simulink model "AMCLStateMachine"  (R2016b)
settings: Solver=FixedStepDiscrete  StartTime=0.0  StopTime=inf  FixedStep=0.01  RelTol=1e-3  EnableMultiTasking=on
settings Model: Creator=CHENJH43  LastModifiedBy=CHENJH43
settings SolverCC: AutoInsertRateTranBlk=on
settings DataIOCC: LimitDataPoints=on
settings OptimizationCC: LifeSpan=inf
settings DebuggingCC: AllowSymbolicDim=off  SFUnexpectedBacktrackingDiag=warning  SFNoUnconditionalDefaultTransitionDiag=warning  SFExecutionAtInitializationDiag=none
settings GRTTargetCC: TargetLangStandard=C89/C90 (ANSI)  GeneratePreprocessorConditionals=Disable all
settings ConfigComp: CovMetricSettings=dw  CovHtmlReporting=on  CovSaveCumulativeToWorkspaceVar=on  CovSaveSingleToWorkspaceVar=on  CovExternalEMLEnable=off  CovSFcnEnable=off

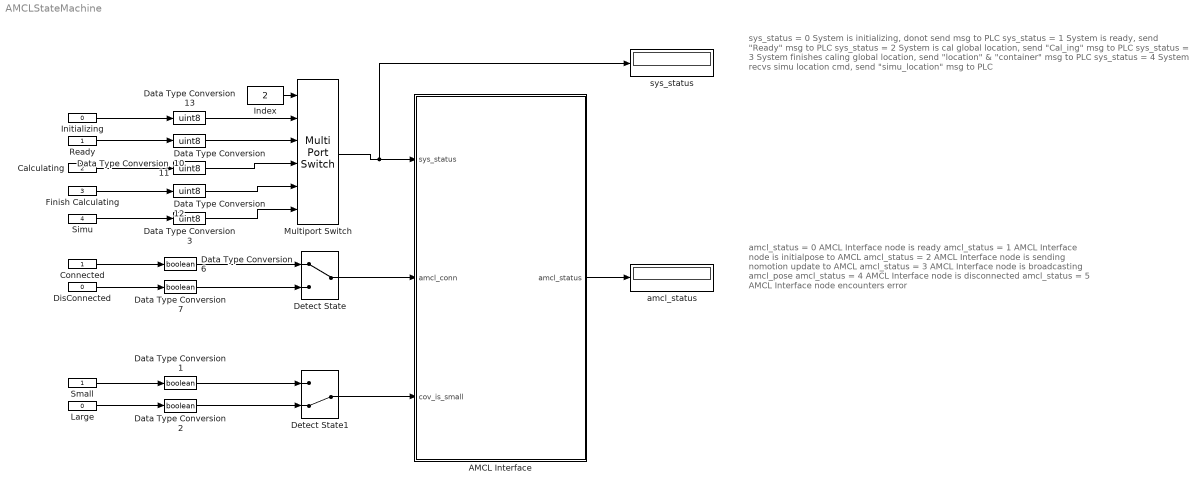
== system AMCLStateMachine ==
  note: amcl_status = 0 AMCL Interface node is ready
      | amcl_status = 1 AMCL Interface node is initialpose to AMCL
      | amcl_status = 2 AMCL Interface node is sending nomotion update to AMCL
      | amcl_status = 3 AMCL Interface node is broadcasting amcl_pose
      | amcl_status = 4 AMCL Interface node is disconnected
      | amcl_status = 5 AMCL Interface node encounters error
  note: sys_status = 0	System is initializing, donot send msg to PLC
      | sys_status = 1	System is ready, send "Ready" msg to PLC
      | sys_status = 2	System is cal global location, send "Cal_ing" msg to PLC
      | sys_status = 3	System finishes caling global location, send "location" & "container" msg to PLC
      | sys_status = 4	System recvs simu location cmd, send "simu_location" msg to PLC
  AMCL Interface : Subsystem
  Calculating : Constant  Value=2
  Connected : Constant
  Data Type Conversion{1..2,6..7} (4 alike) : DataTypeConversion  OutDataTypeStr=boolean
  Data Type Conversion{3,10..13} (5 alike) : DataTypeConversion  OutDataTypeStr=uint8
  Detect State : ManualSwitch
  Detect State1 : ManualSwitch  CurrentSetting=0
  DisConnected : Constant  Value=0
  Finish Calculating : Constant  Value=3
  Index : Constant  Value=2
  Initializing : Constant  Value=0
  Large : Constant  Value=0
  Multiport Switch : MultiPortSwitch  DataPortOrder=Zero-based contiguous  Inputs=5
  Ready : Constant
  Simu : Constant  Value=4
  Small : Constant
  amcl_status : Display
  sys_status : Display
  wires:
  Calculating/1 -> Data Type Conversion11/1
  Finish Calculating/1 -> Data Type Conversion12/1
  Data Type Conversion11/1 -> Multiport Switch/4
  Data Type Conversion12/1 -> Multiport Switch/5
  Ready/1 -> Data Type Conversion10/1
  Initializing/1 -> Data Type Conversion13/1
  Data Type Conversion10/1 -> Multiport Switch/3
  Data Type Conversion13/1 -> Multiport Switch/2
  Connected/1 -> Data Type Conversion6/1
  DisConnected/1 -> Data Type Conversion7/1
  Data Type Conversion6/1 -> Detect State/1
  Data Type Conversion7/1 -> Detect State/2
  Small/1 -> Data Type Conversion1/1
  Large/1 -> Data Type Conversion2/1
  Data Type Conversion1/1 -> Detect State1/1
  Data Type Conversion2/1 -> Detect State1/2
  Simu/1 -> Data Type Conversion3/1
  Data Type Conversion3/1 -> Multiport Switch/6
  Multiport Switch/1 -> sys_status/1, AMCL Interface/1(sys_status)
  Detect State/1 -> AMCL Interface/2(amcl_conn)
  Detect State1/1 -> AMCL Interface/3(cov_is_small)
  AMCL Interface/1(amcl_status) -> amcl_status/1
  Index/1 -> Multiport Switch/1

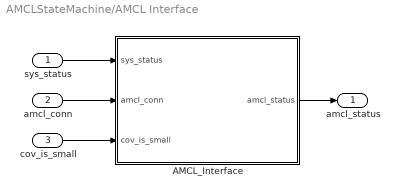
== system AMCLStateMachine/AMCL Interface ==
  sys_status : Inport
  amcl_conn : Inport  Port=2
  cov_is_small : Inport  Port=3
  AMCL_Interface : Stateflow chart  TreatAsAtomicUnit=on
  amcl_status : Outport
  wires:
  AMCL_Interface/1(amcl_status) -> amcl_status/1
  sys_status/1 -> AMCL_Interface/1(sys_status)
  amcl_conn/1 -> AMCL_Interface/2(amcl_conn)
  cov_is_small/1 -> AMCL_Interface/3(cov_is_small)

== stateflow chart AMCLStateMachine/AMCL Interface/AMCL_Interface ==
  settings: updateMethod=DISCRETE  sampleTime=0.01
  state AMCLReady
    during:amcl_status = 0;
  state SendInitPose
    entry:send_count = 0;
    during:amcl_status = 1;
    during:send_count  = send_count + 1;
  state AMCLDisconn
    during:amcl_status = 4;
  state SendToughLocation
    during:amcl_status = 3;
  state UpdatePose
    entry:update_count = 0;
    during:amcl_status = 2;
    during:update_count = update_count + 1;
  state Error
    during:amcl_status = 5;
  AMCLReady -> (junction 20) [order 2] : [sys_status == 2]
  (junction 20) -> SendInitPose : {init_count = 0}
  Error -> AMCLReady
  SendInitPose -> AMCLReady [order 2] : [sys_status != 2]
  SendToughLocation -> AMCLReady [order 2] : [sys_status != 2]
  AMCLReady -> AMCLDisconn [order 1] : [amcl_conn == 0]
  AMCLDisconn -> AMCLReady : [amcl_conn == 1]
  SendInitPose -> AMCLDisconn [order 1] : [amcl_conn == 0]
  UpdatePose -> SendInitPose [order 4] : [cov_is_small == 1]
  SendInitPose -> (junction 24) [order 3] : [send_count >= 3 ]
  (default) -> AMCLDisconn
  UpdatePose -> AMCLDisconn [order 1] : [amcl_conn == 0]
  (junction 24) -> UpdatePose : {init_count = init_count + 1}
  SendToughLocation -> AMCLDisconn [order 1] : [amcl_conn == 0]
  UpdatePose -> SendToughLocation [order 3] : [init_count >= 2 && cov_is_small == 1]
  UpdatePose -> Error [order 2] : [update_count > 200]
  data: sys_status input uint8; amcl_conn input boolean; amcl_status output uint8; cov_is_small input boolean; init_count local uint16; send_count local uint16; update_count local uint16
